simulink model "Adder_Cin_1"  (R2018a)
settings: Solver=VariableStepAuto  StartTime=0.0  StopTime=10.0  RelTol=1e-3
settings Model: Creator=midog  LastModifiedBy=midog

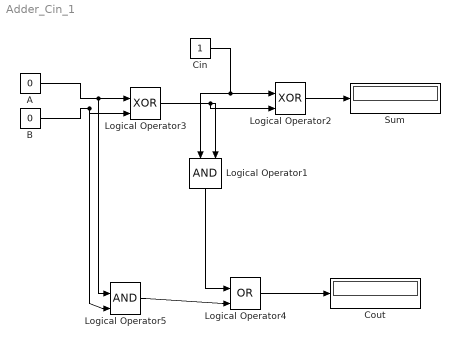
== system Adder_Cin_1 ==
  A : Constant  Value=0
  B : Constant  Value=0
  Cin : Constant
  Cout : Display
  Logical Operator1 : Logic  IconShape=distinctive  AllPortsSameDT=off  OutDataTypeStr=boolean
  Logical Operator2 : Logic  Operator=XOR  IconShape=distinctive  AllPortsSameDT=off  OutDataTypeStr=boolean
  Logical Operator3 : Logic  Operator=XOR  IconShape=distinctive  AllPortsSameDT=off  OutDataTypeStr=boolean
  Logical Operator4 : Logic  Operator=OR  IconShape=distinctive  AllPortsSameDT=off  OutDataTypeStr=boolean
  Logical Operator5 : Logic  IconShape=distinctive  AllPortsSameDT=off  OutDataTypeStr=boolean
  Sum : Display
  wires:
  Cin/1 -> Logical Operator1/1, Logical Operator2/1
  Logical Operator2/1 -> Sum/1
  B/1 -> Logical Operator5/2, Logical Operator3/2
  A/1 -> Logical Operator5/1, Logical Operator3/1
  Logical Operator3/1 -> Logical Operator2/2, Logical Operator1/2
  Logical Operator1/1 -> Logical Operator4/1
  Logical Operator4/1 -> Cout/1
  Logical Operator5/1 -> Logical Operator4/2
